simulink model "HeliDraft_26_02_2025"  (R2024b)
settings: Solver=VariableStepAuto  StartTime=0.0  StopTime=10.0  RelTol=1e-3
values from neighbouring files (symbols this model uses):
  R = D/2    (= 2.01773704722)    [untitled.m]
undefined symbols (not defined in the file or in its folder): Afin, AngVel, AngVeltr, BatteryCap, BatteryDischrgRate, Earth, EngPowSL, Ion, Lfin, Lithium, MTOW, Preq2RPM, RPM2Vreq, WGS84
libraries: fl_lib x7, nesl_utility x5, simulink_extras x4, aerolibatmos2 x2, aerolibanimutils x2, aerolibfltsims x2, aerolibtransform2 x1, shared6dof x1, batteryecm_lib x1, spsBatteryLib x1, spsControlledCurrentSourceLib x1, spspowerguiLib x1
(part 2 of 2)

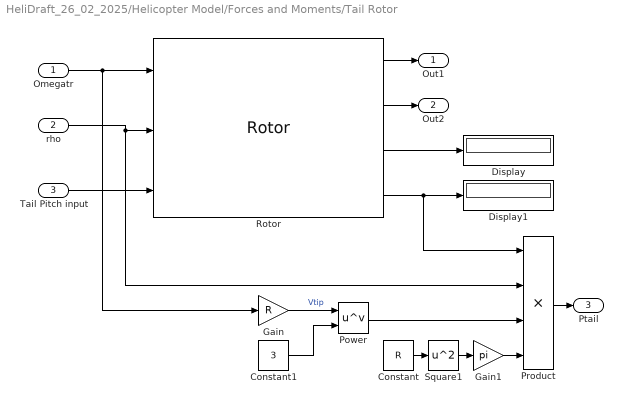
== system HeliDraft_26_02_2025/Helicopter Model/Forces and Moments/Tail Rotor ==
  Omegatr : Inport
  rho : Inport  Port=2
  Tail Pitch input : Inport  Port=3
  Constant : Constant  Value=R
  Constant1 : Constant  Value=3
  Display : Display
  Display1 : Display
  Gain : Gain  Gain=R
  Gain1 : Gain  Gain=pi
  Power : Math  Operator=pow
  Product : Product  Inputs=4
  Rotor : Rotor  controlInput=on  CTCQMode=Compute using BEMT  Nb=Nbtr  CTout=on  radius=Rtr  clalpha=CLalphaTR  cd0=0.009  thetaRoot=0  thetaTwist=0
  Square1 : Math  Operator=square
  Out1 : Outport
  Out2 : Outport  Port=2
  Ptail : Outport  Port=3
  wires:
  Rotor/2 -> Out2/1
  Rotor/1 -> Out1/1
  Rotor/3 -> Display/1
  Tail Pitch input/1 -> Rotor/3
  Power/1 -> Product/3
  Constant1/1 -> Power/2
  Gain/1 -> Power/1  "Vtip"
  rho/1 -> Product/2, Rotor/2
  Rotor/4 -> Product/1, Display1/1
  Gain1/1 -> Product/4
  Omegatr/1 -> Gain/1, Rotor/1
  Square1/1 -> Gain1/1
  Constant/1 -> Square1/1
  Product/1 -> Ptail/1

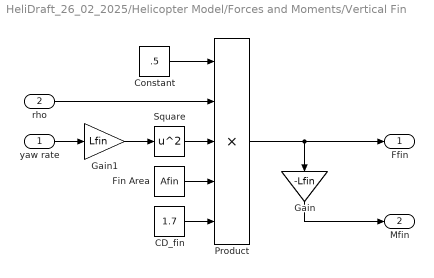
== system HeliDraft_26_02_2025/Helicopter Model/Forces and Moments/Vertical Fin ==
  yaw rate : Inport
  rho : Inport  Port=2
  CD_fin : Constant  Value=1.7
  Constant : Constant  Value=.5
  Fin Area : Constant  Value=Afin
  Gain : Gain  Gain=-Lfin
  Gain1 : Gain  Gain=Lfin
  Product : Product  Inputs=5
  Square : Math  Operator=square
  Ffin : Outport
  Mfin : Outport  Port=2
  wires:
  Product/1 -> Ffin/1, Gain/1
  yaw rate/1 -> Gain1/1
  rho/1 -> Product/2
  Constant/1 -> Product/1
  Gain1/1 -> Square/1
  Square/1 -> Product/3
  Fin Area/1 -> Product/4
  CD_fin/1 -> Product/5
  Gain/1 -> Mfin/1

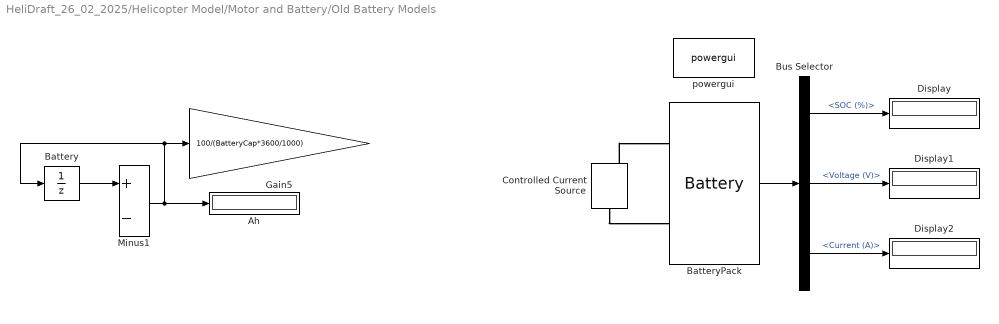
== system HeliDraft_26_02_2025/Helicopter Model/Motor and Battery/Old Battery Models ==
  Ah : Display
      settings: Format=bank
  Battery : UnitDelay  InitialCondition=BatteryCap*3600/1000  HasFrameUpgradeWarning=on
  BatteryPack : spsBatteryLib/Battery  BatType=Lithium-Ion  NomV=BatteryVnom  NomQ=BatteryCap/1000  SOC=100  Batt_Tr=30  PresetModel=on  MaxQ=140  MinV=5.4  FullV=7.8395  Dis_rate=60.8696  R=0.013333  Normal_OP=126.6087  expZone="[151.254      6.878261]"
  Bus Selector : BusSelector  OutputSignals=SOC (%),Voltage (V),Current (A)
  Controlled Current Source : spsControlledCurrentSourceLib/Controlled Current Source  Initialize=off  Source_Type=DC  Amplitude=66.6  Phase=0  Frequency=0  Measurements=None
  Display : Display
  Display1 : Display
  Display2 : Display
  Gain5 : Gain  Gain=100/(BatteryCap*3600/1000)
  Minus1 : Sum  Inputs=+-
  powergui : spspowerguiLib/powergui  Priority=1  SimulationMode=Continuous  SampleTime=50e-6  frequency=60  Iterations=50  frequencyindice=0  Pbase=100e6  ErrMax=1e-4  UnitsV=kV  UnitsW=MW  buscounter=0  FunctionMessages=off  echomessages=off  EnableUseOfTLC=off  CurrentSourceSwitches=off  DisableSnubberDevices=off  DisableRonSwitches=off  DisableVfSwitches=off  DisplayEquations=off  AutomaticDiscreteSolvers=off  SolverType=Tustin/Backward Euler (TBE)  Interpol=off  ExternalGateDelay=off  methode=off  Ts=100  x0status=blocks  SPID=on  SwTol=0  HookPort=off  NonlinearTolerance=1e-4  nMaxIteration=100  ContinueOnMaxIteration=off  RestoreLinks=warning  ResistiveCurrentMeasurement=off  Frange=[0:2:500]  Ylog=off  Xlog=on  ShowGrid=off  save=off  variable=ZData  structure=0  ZoomFFT=off  StartTime=0.0  cycles=1  DisplayStyle=1  fundamental=60  FreqAxis=off  MaxFrequency=1000  frequencyindicesteady=1  RmsSteady=1  display=off
  wires:
  Minus1/1 -> Battery/1, Gain5/1, Ah/1
  Battery/1 -> Minus1/1
  Bus Selector/3 -> Display2/1  "<Current (A)>"
  BatteryPack/1 -> Bus Selector/1
  Bus Selector/2 -> Display1/1  "<Voltage (V)>"
  Bus Selector/1 -> Display/1  "<SOC (%)>"
  connections:
  Controlled Current Source/LConn1 -- BatteryPack/LConn1
  Controlled Current Source/RConn1 -- BatteryPack/LConn2
